simulink library "db_"  (R2014b)
settings: Solver=ode45  SolverMode=SingleTasking  StartTime=0.0  StopTime=10.0  RelTol=1e-3
values from neighbouring files (symbols this model uses):
  B1 = 40    [ejemplo_mecanico.m]    (also in veengranes.m = 10)
  B2 = 20    [ejemplo_mecanico.m]    (also in veengranes.m = 34)
  J1 = 200    [Problem_5_Matlab.m]    (also in grupo_roberto.m = 3; veengranes.m = 2)
  J2 = 10    [Problem_5_Matlab.m]    (also in grupo_roberto.m = 3; veengranes.m = 4)
  K1 = 700    [Problem_5_Matlab.m]    (also in ejemplo_mecanico.m = 100; ejercicio7_taller2SM.m = 34; grupo_roberto.m = 3; veengranes.m = 5)
  K2 = 20    [Problem_5_Matlab.m]    (also in ejercicio7_taller2SM.m = 300; grupo_roberto.m = 3; veengranes.m = 4)
  r1 = 0.5    [veengranes.m]
  r2 = 0.1    [veengranes.m]
settings Model: CovMetricSettings=dwe  CovHtmlReporting=off  CovSaveCumulativeToWorkspaceVar=off  CovSaveSingleToWorkspaceVar=off  CovExternalEMLEnable=on  CovSFcnEnable=on  Creator=carma  LastModifiedBy=carma

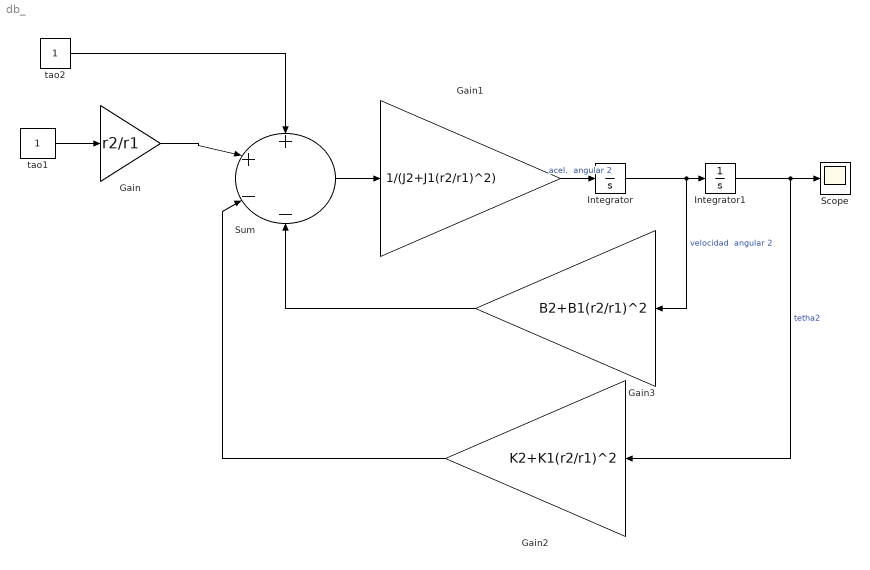
== system db_ ==
  Gain : Gain  Gain=r2/r1
  Gain1 : Gain  Gain=1/(J2+J1(r2/r1)^2)
  Gain2 : Gain  Gain=K2+K1(r2/r1)^2
  Gain3 : Gain  Gain=B2+B1(r2/r1)^2
  Integrator : Integrator
  Integrator1 : Integrator
  Scope : Scope
      settings: TimeRange=auto  MaxDataPoints=5000  SaveToWorkspace=off  SaveName=ScopeData  YMin=-10  YMax=10  SampleTime=-1
  Sum : Sum  Inputs=++--
  tao1 : Constant
  tao2 : Constant
  wires:
  tao2/1 -> Sum/1
  tao1/1 -> Gain/1
  Gain/1 -> Sum/2
  Sum/1 -> Gain1/1
  Gain1/1 -> Integrator/1  "acel.  angular 2"
  Integrator/1 -> Gain3/1, Integrator1/1  "velocidad  angular 2"
  Integrator1/1 -> Gain2/1, Scope/1  "tetha2"
  Gain2/1 -> Sum/3
  Gain3/1 -> Sum/4
